simulink subsystem "rtdSound"  (R2023b)
settings: Solver=VariableStepAuto  StartTime=0.0  StopTime=10.0  RelTol=1e-3
libraries: steeringWheel_lib x1
settings Model: Creator=serga  LastModifiedBy=serga

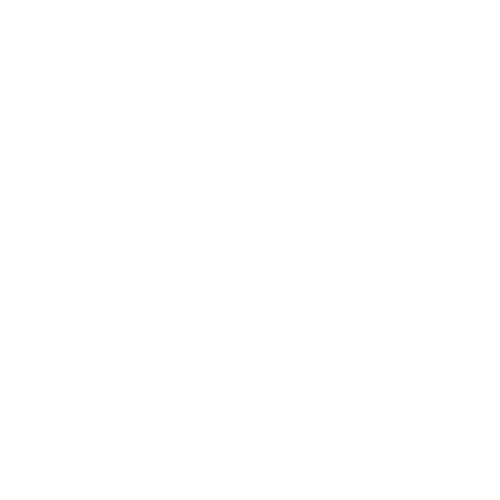
[thumbnail: Simulink's stored preview of the top-level diagram]
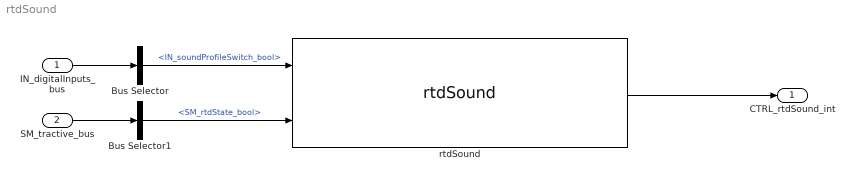
== system rtdSound ==
  IN_digitalInputs_bus : Inport
  SM_tractive_bus : Inport  Port=2
  Bus Selector : BusSelector  OutputSignals=IN_steeringWheel_bus.IN_soundProfileSwitch_bool
  Bus Selector1 : BusSelector  OutputSignals=SM_rtdState_bool
  rtdSound : steeringWheel_lib/rtdSound  SystemSampleTime=-1  VariantActivationTime=update diagram  AllowFlexibleInterface=on  Latency=0  AutoFrameSizeCalculation=off
  CTRL_rtdSound_int : Outport
  wires:
  IN_digitalInputs_bus/1 -> Bus Selector/1
  rtdSound/1 -> CTRL_rtdSound_int/1
  SM_tractive_bus/1 -> Bus Selector1/1
  Bus Selector/1 -> rtdSound/1  "<IN_soundProfileSwitch_bool>"
  Bus Selector1/1 -> rtdSound/2  "<SM_rtdState_bool>"
